simulink model "actividad_01"  (R2021b)
settings: Solver=VariableStepAuto  StartTime=0.0  StopTime=10.0  RelTol=1e-3
libraries: slpidlib x2
settings Model: Creator=osher  LastModifiedBy=osher

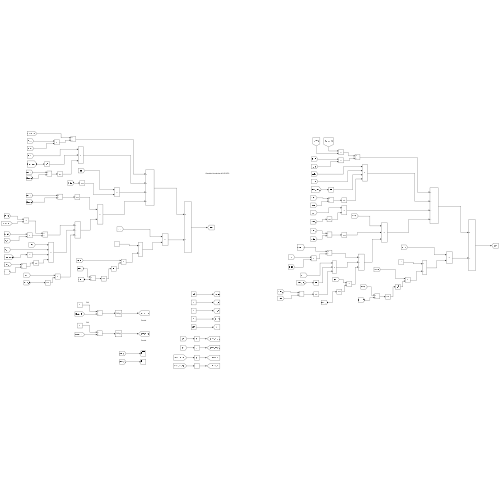
[thumbnail: Simulink's stored preview of the top-level diagram]
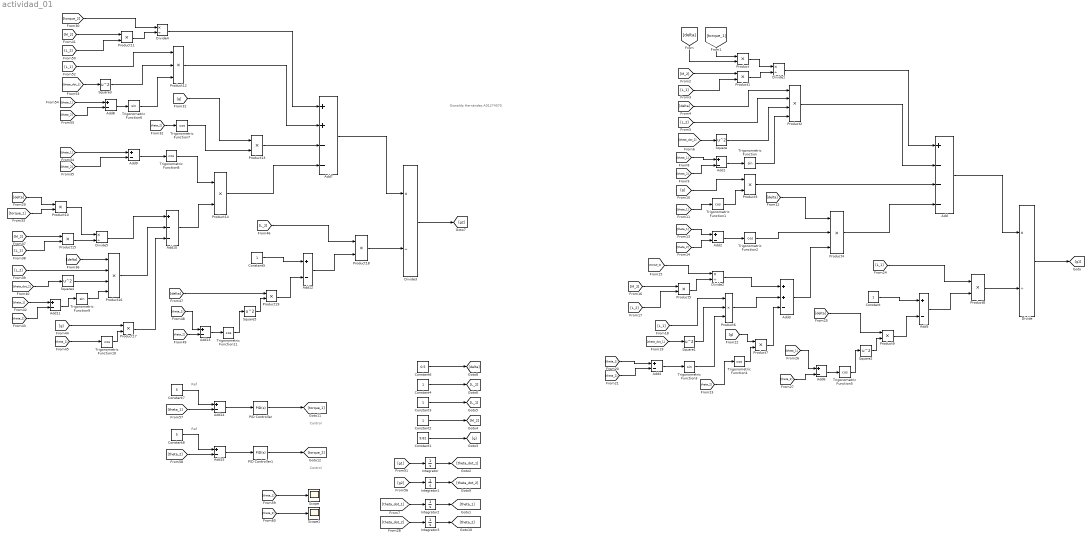
== system actividad_01 ==
  note: Oswaldo Hernández A01274570
  note: Ref
  note: Control
  note: Ref
  note: Control
  Add : Sum  Inputs=+---
  Add{1..2,4..6,8..9,11..15} (12 alike) : Sum  Inputs=+-
  Add10 : Sum  Inputs=+--
  Add3 : Sum  Inputs=++-
  Add7 : Sum  Inputs=++--
  Constant{,2..5} (5 alike) : Constant
  Constant1 : Constant  Value=9.81
  Constant6 : Constant  Value=0.5
  Constant7 : Constant  Value=5
  Constant8 : Constant  Value=5
  Divide{,1..5} (6 alike) : Product  Inputs=*/
  Integrator{,1..3} (4 alike) : Integrator
  PID Controller : slpidlib/PID Controller  Controller=PID  Form=Parallel  TimeDomain=Continuous-time  UseExternalTs=off  SampleTime=-1  IntegratorMethod=Forward Euler  FilterMethod=Forward Euler  ControllerParametersSource=internal  P=418840.989190179  I=29401885.6881851  D=1464.93248323503  UseFilter=on  N=8202.47981765596  TunerSelectOption=Transfer Function Based (PID Tuner App)  InitialConditionSource=internal  InitialConditionForIntegrator=0  InitialConditionForFilter=0  DifferentiatorICPrevScaledInput=0  ExternalReset=none  TrackingMode=off  Kt=1  LimitOutput=off  SatLimitsSource=internal  UpperSaturationLimit=inf  LowerSaturationLimit=-inf  LinearizeAsGain=on  AntiWindupMode=none  Kb=1  POutMin=[]  POutMax=[]  IOutMin=[]  IOutMax=[]  DOutMin=[]  DOutMax=[]  NOutMin=[]  NOutMax=[]  SumOutMin=[]  SumOutMax=[]  SaturationOutMin=[]  SaturationOutMax=[]  PParamMin=[]  PParamMax=[]  IParamMin=[]  IParamMax=[]  DParamMin=[]  DParamMax=[]  NParamMin=[]  NParamMax=[]  KbParamMin=[]  KbParamMax=[]  KtParamMin=[]  KtParamMax=[]  KbOutMin=[]  KbOutMax=[]  KtOutMin=[]  KtOutMax=[]  IntegratorOutMin=[]  IntegratorOutMax=[]  FilterOutMin=[]  FilterOutMax=[]  SumI1OutMin=[]  SumI1OutMax=[]  SumI2OutMin=[]  SumI2OutMax=[]  SumI3OutMin=[]  SumI3OutMax=[]  SumI4OutMin=[]  SumI4OutMax=[]  SumDOutMin=[]  SumDOutMax=[]  DifferentiatorOutMin=[]  DifferentiatorOutMax=[]  FilterDiffOutCoefMin=[]  FilterDiffOutCoefMax=[]  ReciprocalOutMin=[]  ReciprocalOutMax=[]  SumDenOutMin=[]  SumDenOutMax=[]  SumNumOutMin=[]  SumNumOutMax=[]  DivideOutMin=[]  DivideOutMax=[]  UdiffTsProdOutMin=[]  UdiffTsProdOutMax=[]  NTsProdOutMin=[]  NTsProdOutMax=[]  UintegralTsProdOutMin=[]  UintegralTsProdOutMax=[]  UngainTsProdOutMin=[]  UngainTsProdOutMax=[]  IntegratorContinuousStateAttributes=''  IntegratorStateMustResolveToSignalObject=off  IntegratorRTWStateStorageClass=Auto  FilterContinuousStateAttributes=''  FilterStateMustResolveToSignalObject=off  FilterRTWStateStorageClass=Auto  ParallelPVariant=InternalParameters  IdealPVariant=Disabled  IVariant=InternalParameters  DVariant=InternalParameters  IntegratorVariant=Continuous  SatVariant=Disabled  AWVariant=Passthrough  PCopyVariant=Disabled  TRVariant=Disabled  FdbkBlocksVariant=Forward  IdealPFdbkVariant=Disabled  SatFdbkVariant=Disabled  DerivativeFilterVariant=ContFilter  NVariant=InternalParameters  NCopyVariant=Disabled  FilterICVariant=InternalICsFilter  IntegratorICVariant=InternalICs  ExternalResetVariant=Disabled  TRSumVariant=Passthrough  SumFdbkVariant=Disabled  SumVariant=Sum_PID  TsampFilterVariant=InternalTs  TsampNgainVariant=Passthrough  TsampIntegralVariant=Passthrough  ExternalSaturationOutDataTypeStr=Inherit: Same as second input
  PID Controller1 : slpidlib/PID Controller  Controller=PID  Form=Parallel  TimeDomain=Continuous-time  UseExternalTs=off  SampleTime=-1  IntegratorMethod=Forward Euler  FilterMethod=Forward Euler  ControllerParametersSource=internal  P=1598461.12839829  I=292573665.66737  D=1313.90536740946  UseFilter=on  N=6380.40518251869  TunerSelectOption=Transfer Function Based (PID Tuner App)  InitialConditionSource=internal  InitialConditionForIntegrator=0  InitialConditionForFilter=0  DifferentiatorICPrevScaledInput=0  ExternalReset=none  TrackingMode=off  Kt=1  LimitOutput=off  SatLimitsSource=internal  UpperSaturationLimit=inf  LowerSaturationLimit=-inf  LinearizeAsGain=on  AntiWindupMode=none  Kb=1  POutMin=[]  POutMax=[]  IOutMin=[]  IOutMax=[]  DOutMin=[]  DOutMax=[]  NOutMin=[]  NOutMax=[]  SumOutMin=[]  SumOutMax=[]  SaturationOutMin=[]  SaturationOutMax=[]  PParamMin=[]  PParamMax=[]  IParamMin=[]  IParamMax=[]  DParamMin=[]  DParamMax=[]  NParamMin=[]  NParamMax=[]  KbParamMin=[]  KbParamMax=[]  KtParamMin=[]  KtParamMax=[]  KbOutMin=[]  KbOutMax=[]  KtOutMin=[]  KtOutMax=[]  IntegratorOutMin=[]  IntegratorOutMax=[]  FilterOutMin=[]  FilterOutMax=[]  SumI1OutMin=[]  SumI1OutMax=[]  SumI2OutMin=[]  SumI2OutMax=[]  SumI3OutMin=[]  SumI3OutMax=[]  SumI4OutMin=[]  SumI4OutMax=[]  SumDOutMin=[]  SumDOutMax=[]  DifferentiatorOutMin=[]  DifferentiatorOutMax=[]  FilterDiffOutCoefMin=[]  FilterDiffOutCoefMax=[]  ReciprocalOutMin=[]  ReciprocalOutMax=[]  SumDenOutMin=[]  SumDenOutMax=[]  SumNumOutMin=[]  SumNumOutMax=[]  DivideOutMin=[]  DivideOutMax=[]  UdiffTsProdOutMin=[]  UdiffTsProdOutMax=[]  NTsProdOutMin=[]  NTsProdOutMax=[]  UintegralTsProdOutMin=[]  UintegralTsProdOutMax=[]  UngainTsProdOutMin=[]  UngainTsProdOutMax=[]  IntegratorContinuousStateAttributes=''  IntegratorStateMustResolveToSignalObject=off  IntegratorRTWStateStorageClass=Auto  FilterContinuousStateAttributes=''  FilterStateMustResolveToSignalObject=off  FilterRTWStateStorageClass=Auto  ParallelPVariant=InternalParameters  IdealPVariant=Disabled  IVariant=InternalParameters  DVariant=InternalParameters  IntegratorVariant=Continuous  SatVariant=Disabled  AWVariant=Passthrough  PCopyVariant=Disabled  TRVariant=Disabled  FdbkBlocksVariant=Forward  IdealPFdbkVariant=Disabled  SatFdbkVariant=Disabled  DerivativeFilterVariant=ContFilter  NVariant=InternalParameters  NCopyVariant=Disabled  FilterICVariant=InternalICsFilter  IntegratorICVariant=InternalICs  ExternalResetVariant=Disabled  TRSumVariant=Passthrough  SumFdbkVariant=Disabled  SumVariant=Sum_PID  TsampFilterVariant=InternalTs  TsampNgainVariant=Passthrough  TsampIntegralVariant=Passthrough  ExternalSaturationOutDataTypeStr=Inherit: Same as second input
  Product{,1,3,5,7..11,13..15,17..19} (15 alike) : Product
  Product12 : Product  Inputs=3
  Product16 : Product  Inputs=4
  Product2 : Product  Inputs=4
  Product4 : Product  Inputs=3
  Product6 : Product  Inputs=3
  Scope : Scope
  Scope1 : Scope
  Square{,1..5} (6 alike) : Math  Operator=square  SaturateOnIntegerOverflow=on
  Trigonometric Function{,3,6,9} (4 alike) : Trigonometry
  Trigonometric Function{1..2,4..5,7..8,10..11} (8 alike) : Trigonometry  Operator=cos
  wires:
  Divide/1 -> [g1]
  Add/1 -> Divide/1
  Divide1/1 -> Add/1
  [torque_1] -> Product/1
  [delta] -> Product/2
  Product/1 -> Divide1/1
  [L_1] -> Product1/2
  [M_2] -> Product1/1
  Product1/1 -> Divide1/2
  Product2/1 -> Add/2
  [delta] -> Product2/1
  [L_2] -> Product2/2
  [theta_dot_2] -> Square/1
  Square/1 -> Product2/3
  [theta_1] -> Add1/1
  [theta_2] -> Add1/2
  Add1/1 -> Trigonometric Function/1
  Trigonometric Function/1 -> Product2/4
  [g] -> Product3/1
  [theta_1] -> Trigonometric Function1/1
  Trigonometric Function1/1 -> Product3/2
  Product3/1 -> Add/3
  Product4/1 -> Add/4
  [delta] -> Product4/1
  [theta_1] -> Add2/1
  [theta_2] -> Add2/2
  Add2/1 -> Trigonometric Function2/1
  Trigonometric Function2/1 -> Product4/2
  Add3/1 -> Product4/3
  [torque_2] -> Divide2/1
  Divide2/1 -> Add3/1
  Product5/1 -> Divide2/2
  [M_2] -> Product5/1
  [L_2] -> Product5/2
  Product6/1 -> Add3/2
  [L_1] -> Product6/1
  [theta_dot_1] -> Square1/1
  Square1/1 -> Product6/2
  Trigonometric Function3/1 -> Product6/3
  Add4/1 -> Trigonometric Function3/1
  [theta_2] -> Add4/2
  [theta_1] -> Add4/1
  Product7/1 -> Add3/3
  [g] -> Product7/1
  Trigonometric Function4/1 -> Product7/2
  [theta_2] -> Trigonometric Function4/1
  Product8/1 -> Divide/2
  [L_1] -> Product8/1
  Constant/1 -> Add5/1
  Add5/1 -> Product8/2
  Product9/1 -> Add5/2
  [delta] -> Product9/1
  Trigonometric Function5/1 -> Square2/1
  Square2/1 -> Product9/2
  Add6/1 -> Trigonometric Function5/1
  [theta_1] -> Add6/1
  [theta_2] -> Add6/2
  Constant1/1 -> [g]
  Constant2/1 -> [M_2]
  Constant3/1 -> [L_1]
  Constant4/1 -> [L_2]
  Trigonometric Function8/1 -> Product14/1
  [theta_2] -> Add13/2
  [theta_1] -> Add9/1
  Add9/1 -> Trigonometric Function8/1
  Add12/1 -> Product18/2
  Product17/1 -> Add10/3
  [theta_2] -> Add9/2
  Product19/1 -> Add12/2
  [L_2] -> Product18/1
  Trigonometric Function10/1 -> Product17/2
  Product14/1 -> Add7/4
  Product16/1 -> Add10/2
  [theta_1] -> Trigonometric Function10/1
  [theta_1] -> Add11/1
  [L_1] -> Product15/2
  [theta_1] -> Add13/1
  [torque_2] -> Divide4/1
  [M_2] -> Product11/1
  [L_1] -> Product12/1
  [theta_2] -> Add11/2
  Product11/1 -> Divide4/2
  Square5/1 -> Product19/2
  [theta_2] -> Trigonometric Function7/1
  [theta_1] -> Add8/1
  Product12/1 -> Add7/2
  Square3/1 -> Product12/2
  Divide4/1 -> Add7/1
  Divide3/1 -> [g2]
  [L_2] -> Product16/2
  Add7/1 -> Divide3/1
  Add13/1 -> Trigonometric Function11/1
  Product18/1 -> Divide3/2
  Product13/1 -> Add7/3
  [theta_2] -> Add8/2
  [delta] -> Product19/1
  [g] -> Product13/1
  Trigonometric Function7/1 -> Product13/2
  [theta_dot_2] -> Square4/1
  Divide5/1 -> Add10/1
  Product15/1 -> Divide5/2
  Square4/1 -> Product16/3
  [M_2] -> Product15/1
  Trigonometric Function11/1 -> Square5/1
  [g] -> Product17/1
  Constant5/1 -> Add12/1
  [L_2] -> Product11/2
  [theta_dot_1] -> Square3/1
  Add11/1 -> Trigonometric Function9/1
  Trigonometric Function9/1 -> Product16/4
  Add8/1 -> Trigonometric Function6/1
  Trigonometric Function6/1 -> Product12/3
  Add10/1 -> Product14/2
  [delta] -> Product10/1
  [torque_1] -> Product10/2
  Product10/1 -> Divide5/1
  [delta] -> Product16/1
  Constant6/1 -> [delta]
  [g1] -> Integrator/1
  Integrator/1 -> [theta_dot_1]
  [g2] -> Integrator1/1
  Integrator1/1 -> [theta_dot_2]
  [theta_dot_1] -> Integrator2/1
  Integrator2/1 -> [theta_1]
  [theta_dot_2] -> Integrator3/1
  Integrator3/1 -> [theta_2]
  PID Controller/1 -> [torque_1]
  Add14/1 -> PID Controller/1
  Constant7/1 -> Add14/1
  [theta_1] -> Add14/2
  Add15/1 -> PID Controller1/1
  [theta_2] -> Add15/2
  PID Controller1/1 -> [torque_2]
  Constant8/1 -> Add15/1
  [theta_1] -> Scope/1
  [theta_2] -> Scope1/1
